simulink model "project_simulink"  (R2022b)
settings: Solver=ode45  StartTime=0.0  StopTime=5  MaxStep=0.2  RelTol=1e-3
values from neighbouring files (symbols this model uses):
  A_cl = A-B*K    [project.m]
  A_obs = A-L*C    [project.m]
  B_obs = [B L]    [project.m]
  C_obs = eye(4)    [project.m]
  D_obs = [D D D D D]    [project.m]
  g = 9.81    [project.m]
  Jb = 0.5 * mb * l^2    (= 0.00014975625)    [project.m]
  Jw = 0.5 * mw * R^2    (= 2.100875e-05)    [project.m]
  l = 0.035    [project.m]
  mb = 0.2445    [project.m]
  mw = 0.0343    [project.m]
  R = 0.035    [project.m]
undefined symbols (not defined in the file or in its folder): A_ol, B_ol, C_ol, D_ol, K_cl
settings Model: Creator=artur  LastModifiedBy=artur
settings SolverCC: MaxConsecutiveMinStep=1000

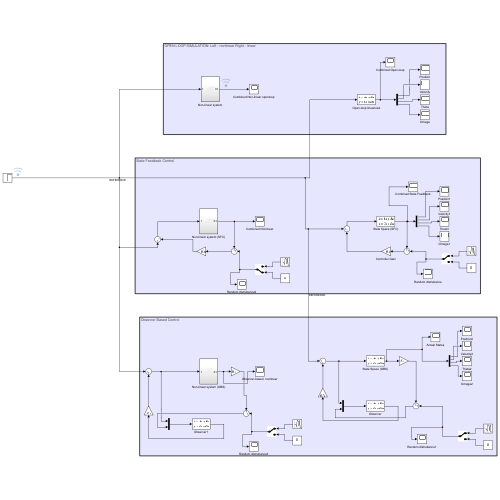
[thumbnail: Simulink's stored preview of the top-level diagram]
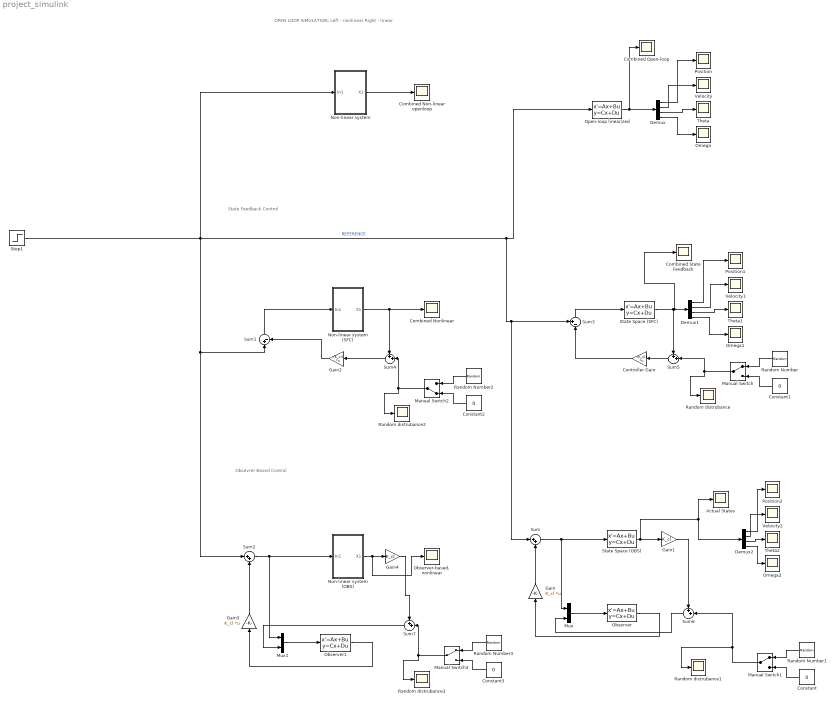
== system project_simulink ==
  note: Obsevrer Based Control
  note: State Feedback Control
  note: OPEN LOOP SIMULATION: Left - nonlinear Right - linear
  Actual States : Scope
  Combined Non-linear openloop : Scope
  Combined Nonlinear : Scope
  Combined Open-loop : Scope
  Combined State Feedback : Scope
  Constant{,1..3} (4 alike) : Constant  Value=0
  Controller Gain : Gain  Gain=(K_cl)  Multiplication=Matrix(K*u)
  Demux : Demux
  Demux1 : Demux
  Demux2 : Demux
  Gain : Gain  Gain=K_cl  Multiplication=Matrix(K*u)
  Gain1 : Gain  Gain=K_cl
  Gain2 : Gain  Gain=(K_cl)  Multiplication=Matrix(K*u)
  Gain3 : Gain  Gain=K_cl  Multiplication=Matrix(K*u)
  Gain4 : Gain  Gain=K_cl
  Manual Switch : ManualSwitch
  Manual Switch1 : ManualSwitch
  Manual Switch2 : ManualSwitch  CurrentSetting=0
  Manual Switch3 : ManualSwitch
  Mux : Mux  Inputs=2
  Mux1 : Mux  Inputs=2
  Non-linear system : Subsystem
  Non-linear system (OBS) : Subsystem
  Non-linear system (SFC) : Subsystem
  Observer : StateSpace  A=A_obs  B=B_obs  C=C_obs  D=D_obs  InitialCondition=0
  "Observer-based, nonlinear" : Scope
  Observer1 : StateSpace  A=A_obs  B=B_obs  C=C_obs  D=D_obs  InitialCondition=0
  Omega : Scope
  Omega1 : Scope
  Omega2 : Scope
  Open-loop linearized : StateSpace  A=A_ol  B=B_ol  C=C_ol  D=D_ol  InitialCondition=0
  Position : Scope
  Position1 : Scope
  Position2 : Scope
  Random Number : RandomNumber  SampleTime=1.5
  Random Number1 : RandomNumber  SampleTime=2
  Random Number2 : RandomNumber  SampleTime=1.5
  Random Number3 : RandomNumber  SampleTime=1.5
  Random distrubance{,1..3} (4 alike) : Scope
  State Space (OBS) : StateSpace  A=A_cl  B=B_ol  C=C_ol  D=D_ol  InitialCondition=0
  State Space (SFC) : StateSpace  A=A_ol  B=B_ol  C=C_ol  D=D_ol  InitialCondition=0  ParameterTunability=Unconstrained
  Step1 : Step  Time=0  SampleTime=0
  Sum : Sum  Inputs=|++
  Sum1 : Sum  Inputs=|+-
  Sum2 : Sum  Inputs=|++
  Sum3 : Sum  Inputs=+-|
  Sum{4..7} (4 alike) : Sum  Inputs=++|
  Theta : Scope
  Theta1 : Scope
  Theta2 : Scope
  Velocity : Scope
  Velocity1 : Scope
  Velocity2 : Scope
  wires:
  Open-loop linearized/1 -> Demux/1, Combined Open-loop/1
  Demux/1 -> Position/1
  Demux/2 -> Velocity/1
  Demux/3 -> Theta/1
  Demux/4 -> Omega/1
  Demux1/4 -> Omega1/1
  Demux1/3 -> Theta1/1
  Demux1/2 -> Velocity1/1
  Demux1/1 -> Position1/1
  State Space (SFC)/1 -> Combined State Feedback/1, Demux1/1, Sum5/1
  State Space (OBS)/1 -> Actual States/1, Demux2/1, Gain1/1
  Demux2/1 -> Position2/1
  Demux2/2 -> Velocity2/1
  Demux2/3 -> Theta2/1
  Demux2/4 -> Omega2/1
  Mux/1 -> Observer/1
  Sum/1 -> Mux/1, State Space (OBS)/1
  Observer/1 -> Gain/1
  Gain/1 -> Sum/2
  Non-linear system/1(X1) -> Combined Non-linear openloop/1
  Sum1/1 -> Non-linear system (SFC)/1(In1)
  Gain2/1 -> Sum1/2
  Non-linear system (SFC)/1(X1) -> Sum4/1, Combined Nonlinear/1
  Gain3/1 -> Sum2/2
  Observer1/1 -> Gain3/1
  Step1/1 -> Non-linear system/1(In1), Sum2/1, Sum1/1, Sum3/1, Sum/1, Open-loop linearized/1  "REFERENCE"
  Mux1/1 -> Observer1/1
  Non-linear system (OBS)/1(X1) -> Gain4/1, "Observer-based, nonlinear"/1
  Sum2/1 -> Mux1/1, Non-linear system (OBS)/1(In1)
  Sum3/1 -> State Space (SFC)/1
  Sum5/1 -> Controller Gain/1
  Constant1/1 -> Manual Switch/2
  Random Number/1 -> Manual Switch/1
  Manual Switch/1 -> Random distrubance/1, Sum5/2
  Manual Switch1/1 -> Sum6/2, Random distrubance1/1
  Random Number1/1 -> Manual Switch1/1
  Constant/1 -> Manual Switch1/2
  Gain1/1 -> Sum6/1
  Sum6/1 -> Mux/2
  Controller Gain/1 -> Sum3/2
  Manual Switch2/1 -> Sum4/2, Random distrubance2/1
  Random Number2/1 -> Manual Switch2/1
  Constant2/1 -> Manual Switch2/2
  Sum4/1 -> Gain2/1
  Constant3/1 -> Manual Switch3/2
  Random Number3/1 -> Manual Switch3/1
  Manual Switch3/1 -> Random distrubance3/1, Sum7/2
  Gain4/1 -> Sum7/1
  Sum7/1 -> Mux1/2

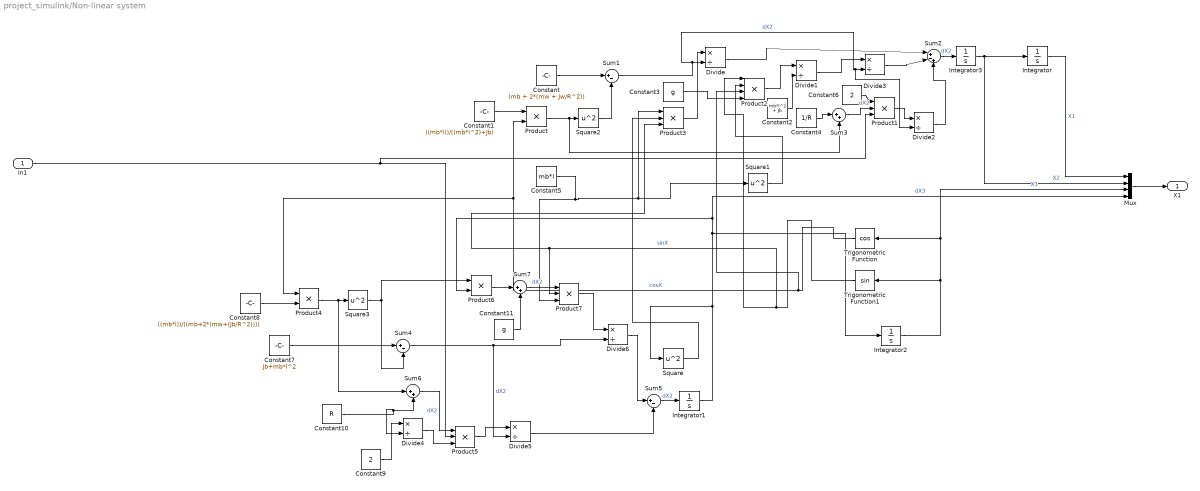
== system project_simulink/Non-linear system ==
  In1 : Inport
  Constant : Constant  Value=(mb + 2*(mw + Jw/R^2))
  Constant1 : Constant  Value=((mb*l))/((mb*l^2)+Jb)
  Constant10 : Constant  Value=R
  Constant11 : Constant  Value=g
  Constant2 : Constant  Value=mb*l^2 + Jb
  Constant3 : Constant  Value=g
  Constant4 : Constant  Value=1/R
  Constant5 : Constant  Value=mb*l
  Constant6 : Constant  Value=2
  Constant7 : Constant  Value=Jb+mb*l^2
  Constant8 : Constant  Value=((mb*l))/((mb+2*(mw+(Jb/R^2))))
  Constant9 : Constant  Value=2
  Divide{,1..6} (7 alike) : Product  Inputs=*/
  Integrator : Integrator  ContinuousStateAttributes='x1'
  Integrator1 : Integrator
  Integrator2 : Integrator
  Integrator3 : Integrator
  Mux : Mux
  Product : Product
  Product{1,3,5,7} (4 alike) : Product  Inputs=3
  Product2 : Product  Inputs=4
  Product4 : Product
  Product6 : Product
  Square{,1..3} (4 alike) : Math  Operator=square
  Sum1 : Sum  Inputs=|+-
  Sum2 : Sum  Inputs=|+-+
  Sum3 : Sum  Inputs=|++
  Sum4 : Sum  Inputs=|+-
  Sum5 : Sum  Inputs=|+-
  Sum6 : Sum  Inputs=|++
  Sum7 : Sum  Inputs=|++
  Trigonometric Function : Trigonometry  Operator=cos
  Trigonometric Function1 : Trigonometry
  X1 : Outport
  wires:
  Constant1/1 -> Product/1
  Product2/1 -> Divide1/1
  Integrator2/1 -> Mux/3, Trigonometric Function/1, Trigonometric Function1/1  "X3"
  Product6/1 -> Sum7/1
  Divide3/1 -> Sum2/2
  Product/1 -> Sum3/2, Square2/1
  Divide4/1 -> Product5/3
  Divide2/1 -> Sum2/3
  Divide6/1 -> Sum5/1
  Sum1/1 -> Divide/2, Divide2/2, Divide3/2  "dX2"
  Constant7/1 -> Sum4/1
  Constant/1 -> Sum1/1
  Trigonometric Function1/1 -> Product2/1, Product7/2, Product3/3  "sinX"
  Integrator1/1 -> Integrator2/1, Mux/4, Product6/2, Square/1  "dX3"
  In1/1 -> Product1/3, Product5/2
  Constant5/1 -> Product7/3, Square1/1, Product3/1
  Constant11/1 -> Sum7/2
  Constant4/1 -> Sum3/1
  Product3/1 -> Divide/1
  Divide/1 -> Sum2/1
  Sum4/1 -> Divide6/2, Divide5/2  "dX2"
  Product4/1 -> Sum6/1, Square3/1
  Product5/1 -> Divide5/1
  Sum2/1 -> Integrator3/1  "dX2"
  Trigonometric Function/1 -> Product2/3, Product4/1, Product/2  "cosX"
  Integrator3/1 -> Mux/2, Integrator/1  "X2"
  Constant10/1 -> Divide4/2, Sum6/2
  Square/1 -> Product3/2
  Square1/1 -> Product2/2
  Sum6/1 -> Product5/1  "dX2"
  Square3/1 -> Product6/1, Sum4/2
  Divide1/1 -> Divide3/1
  Constant6/1 -> Product1/1
  Constant9/1 -> Divide4/1
  Sum7/1 -> Product7/1  "dX2"
  Product1/1 -> Divide2/1
  Sum5/1 -> Integrator1/1  "dX2"
  Square2/1 -> Sum1/2
  Divide5/1 -> Sum5/2
  Constant8/1 -> Product4/2
  Sum3/1 -> Product1/2  "dX2"
  Constant3/1 -> Product2/4
  Constant2/1 -> Divide1/2
  Product7/1 -> Divide6/1
  Mux/1 -> X1/1
  Integrator/1 -> Mux/1  "X1"

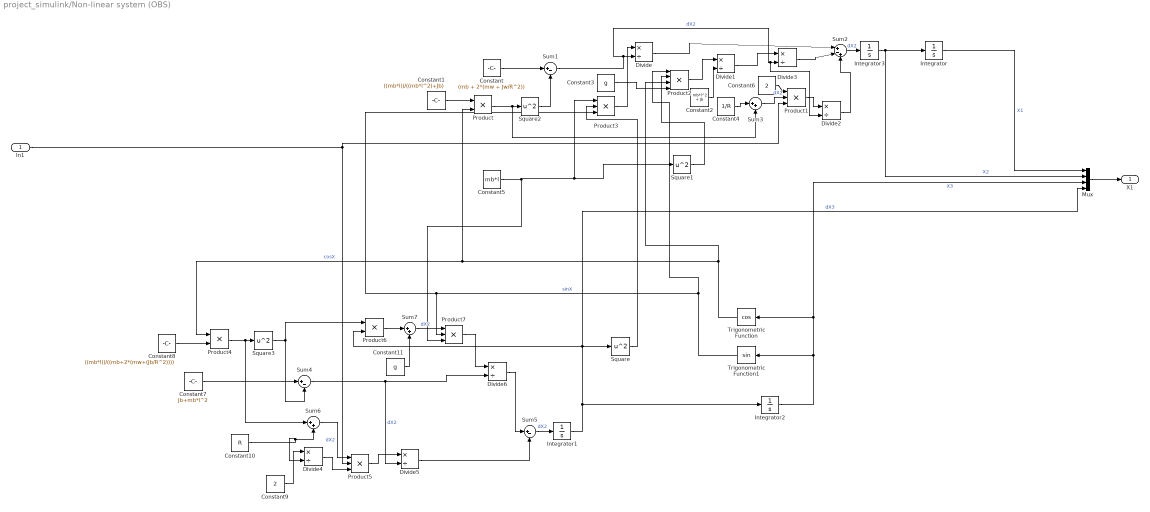
== system project_simulink/Non-linear system (OBS) ==
  In1 : Inport
  Constant : Constant  Value=(mb + 2*(mw + Jw/R^2))
  Constant1 : Constant  Value=((mb*l))/((mb*l^2)+Jb)
  Constant10 : Constant  Value=R
  Constant11 : Constant  Value=g
  Constant2 : Constant  Value=mb*l^2 + Jb
  Constant3 : Constant  Value=g
  Constant4 : Constant  Value=1/R
  Constant5 : Constant  Value=mb*l
  Constant6 : Constant  Value=2
  Constant7 : Constant  Value=Jb+mb*l^2
  Constant8 : Constant  Value=((mb*l))/((mb+2*(mw+(Jb/R^2))))
  Constant9 : Constant  Value=2
  Divide{,1..6} (7 alike) : Product  Inputs=*/
  Integrator : Integrator  ContinuousStateAttributes='x1'
  Integrator1 : Integrator
  Integrator2 : Integrator
  Integrator3 : Integrator
  Mux : Mux
  Product : Product
  Product{1,3,5,7} (4 alike) : Product  Inputs=3
  Product2 : Product  Inputs=4
  Product4 : Product
  Product6 : Product
  Square{,1..3} (4 alike) : Math  Operator=square
  Sum1 : Sum  Inputs=|+-
  Sum2 : Sum  Inputs=|+-+
  Sum3 : Sum  Inputs=|++
  Sum4 : Sum  Inputs=|+-
  Sum5 : Sum  Inputs=|+-
  Sum6 : Sum  Inputs=|++
  Sum7 : Sum  Inputs=|++
  Trigonometric Function : Trigonometry  Operator=cos
  Trigonometric Function1 : Trigonometry
  X1 : Outport
  wires:
  Constant1/1 -> Product/1
  Product2/1 -> Divide1/1
  Integrator2/1 -> Mux/3, Trigonometric Function/1, Trigonometric Function1/1  "X3"
  Product6/1 -> Sum7/1
  Divide3/1 -> Sum2/2
  Product/1 -> Sum3/2, Square2/1
  Divide4/1 -> Product5/3
  Divide2/1 -> Sum2/3
  Divide6/1 -> Sum5/1
  Sum1/1 -> Divide/2, Divide2/2, Divide3/2  "dX2"
  Constant7/1 -> Sum4/1
  Constant/1 -> Sum1/1
  Trigonometric Function1/1 -> Product2/1, Product7/2, Product3/3  "sinX"
  Integrator1/1 -> Mux/4, Product6/2, Square/1, Integrator2/1  "dX3"
  In1/1 -> Product1/3, Product5/2
  Constant5/1 -> Product7/3, Square1/1, Product3/1
  Constant11/1 -> Sum7/2
  Constant4/1 -> Sum3/1
  Product3/1 -> Divide/1
  Divide/1 -> Sum2/1
  Sum4/1 -> Divide6/2, Divide5/2  "dX2"
  Product4/1 -> Sum6/1, Square3/1
  Product5/1 -> Divide5/1
  Sum2/1 -> Integrator3/1  "dX2"
  Trigonometric Function/1 -> Product2/3, Product4/1, Product/2  "cosX"
  Integrator3/1 -> Mux/2, Integrator/1  "X2"
  Constant10/1 -> Divide4/2, Sum6/2
  Square/1 -> Product3/2
  Square1/1 -> Product2/2
  Sum6/1 -> Product5/1  "dX2"
  Square3/1 -> Product6/1, Sum4/2
  Divide1/1 -> Divide3/1
  Constant6/1 -> Product1/1
  Constant9/1 -> Divide4/1
  Sum7/1 -> Product7/1  "dX2"
  Product1/1 -> Divide2/1
  Sum5/1 -> Integrator1/1  "dX2"
  Square2/1 -> Sum1/2
  Divide5/1 -> Sum5/2
  Constant8/1 -> Product4/2
  Sum3/1 -> Product1/2  "dX2"
  Constant3/1 -> Product2/4
  Constant2/1 -> Divide1/2
  Product7/1 -> Divide6/1
  Mux/1 -> X1/1
  Integrator/1 -> Mux/1  "X1"

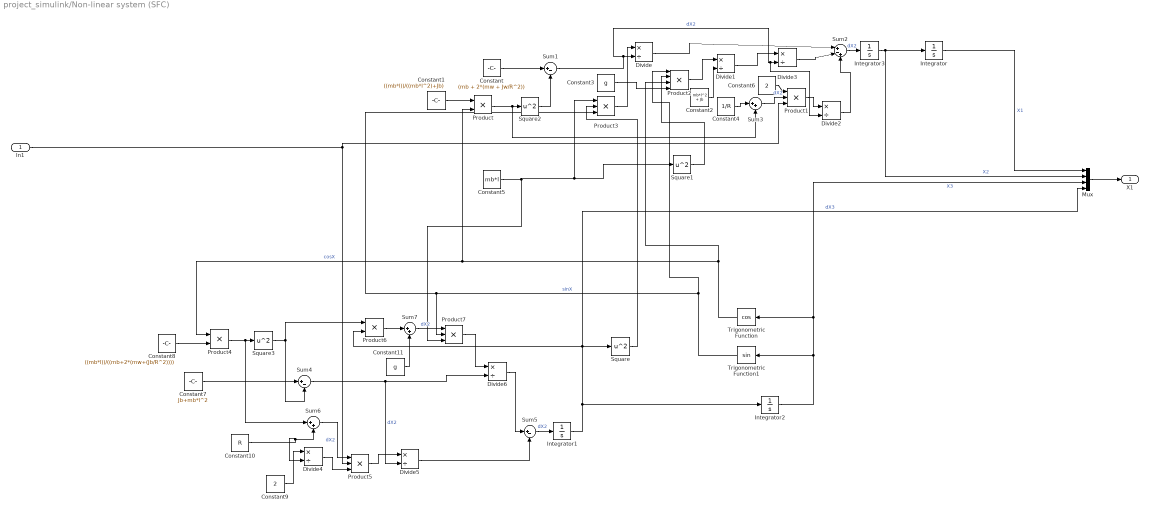
== system project_simulink/Non-linear system (SFC) ==
  In1 : Inport
  Constant : Constant  Value=(mb + 2*(mw + Jw/R^2))
  Constant1 : Constant  Value=((mb*l))/((mb*l^2)+Jb)
  Constant10 : Constant  Value=R
  Constant11 : Constant  Value=g
  Constant2 : Constant  Value=mb*l^2 + Jb
  Constant3 : Constant  Value=g
  Constant4 : Constant  Value=1/R
  Constant5 : Constant  Value=mb*l
  Constant6 : Constant  Value=2
  Constant7 : Constant  Value=Jb+mb*l^2
  Constant8 : Constant  Value=((mb*l))/((mb+2*(mw+(Jb/R^2))))
  Constant9 : Constant  Value=2
  Divide{,1..6} (7 alike) : Product  Inputs=*/
  Integrator : Integrator  ContinuousStateAttributes='x1'
  Integrator1 : Integrator
  Integrator2 : Integrator
  Integrator3 : Integrator
  Mux : Mux
  Product : Product
  Product{1,3,5,7} (4 alike) : Product  Inputs=3
  Product2 : Product  Inputs=4
  Product4 : Product
  Product6 : Product
  Square{,1..3} (4 alike) : Math  Operator=square
  Sum1 : Sum  Inputs=|+-
  Sum2 : Sum  Inputs=|+-+
  Sum3 : Sum  Inputs=|++
  Sum4 : Sum  Inputs=|+-
  Sum5 : Sum  Inputs=|+-
  Sum6 : Sum  Inputs=|++
  Sum7 : Sum  Inputs=|++
  Trigonometric Function : Trigonometry  Operator=cos
  Trigonometric Function1 : Trigonometry
  X1 : Outport
  wires:
  Integrator/1 -> Mux/1  "X1"
  Mux/1 -> X1/1
  Product7/1 -> Divide6/1
  Constant2/1 -> Divide1/2
  Constant3/1 -> Product2/4
  Sum3/1 -> Product1/2  "dX2"
  Constant8/1 -> Product4/2
  Divide5/1 -> Sum5/2
  Square2/1 -> Sum1/2
  Sum5/1 -> Integrator1/1  "dX2"
  Product1/1 -> Divide2/1
  Sum7/1 -> Product7/1  "dX2"
  Constant9/1 -> Divide4/1
  Constant6/1 -> Product1/1
  Divide1/1 -> Divide3/1
  Square3/1 -> Sum4/2, Product6/1
  Sum6/1 -> Product5/1  "dX2"
  Square1/1 -> Product2/2
  Square/1 -> Product3/2
  Constant10/1 -> Sum6/2, Divide4/2
  Integrator3/1 -> Integrator/1, Mux/2  "X2"
  Trigonometric Function/1 -> Product/2, Product4/1, Product2/3  "cosX"
  Sum2/1 -> Integrator3/1  "dX2"
  Product5/1 -> Divide5/1
  Product4/1 -> Square3/1, Sum6/1
  Sum4/1 -> Divide5/2, Divide6/2  "dX2"
  Divide/1 -> Sum2/1
  Product3/1 -> Divide/1
  Constant4/1 -> Sum3/1
  Constant11/1 -> Sum7/2
  Constant5/1 -> Product3/1, Square1/1, Product7/3
  In1/1 -> Product5/2, Product1/3
  Integrator1/1 -> Integrator2/1, Square/1, Product6/2, Mux/4  "dX3"
  Trigonometric Function1/1 -> Product3/3, Product7/2, Product2/1  "sinX"
  Constant/1 -> Sum1/1
  Constant7/1 -> Sum4/1
  Sum1/1 -> Divide3/2, Divide2/2, Divide/2  "dX2"
  Divide6/1 -> Sum5/1
  Divide2/1 -> Sum2/3
  Divide4/1 -> Product5/3
  Product/1 -> Square2/1, Sum3/2
  Divide3/1 -> Sum2/2
  Product6/1 -> Sum7/1
  Integrator2/1 -> Trigonometric Function1/1, Trigonometric Function/1, Mux/3  "X3"
  Product2/1 -> Divide1/1
  Constant1/1 -> Product/1
